simulink model "LQR_with_tracking"  (R2025b)
settings: Solver=ode45  StartTime=0.0  StopTime=Tend  MaxStep=1e-3  MinStep=1e-4  RelTol=1e-3
undefined symbols (not defined in the file): C, DiscIntNeverNeededParam, Kq, Kx, Ts
libraries: cstblocks x1
settings Model: Creator=davidecovolo  LastModifiedBy=davidecovolo
settings SolverCC: InitialStep=1e-4

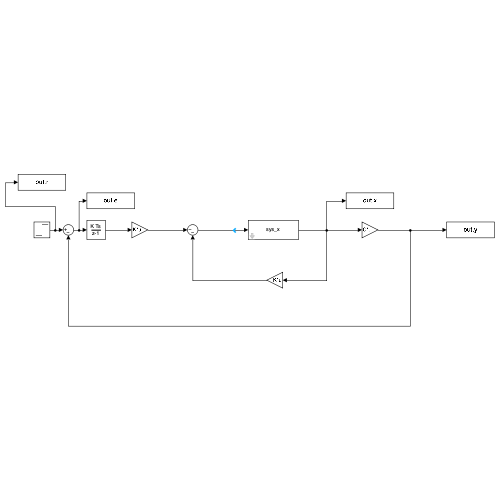
[thumbnail: Simulink's stored preview of the top-level diagram]
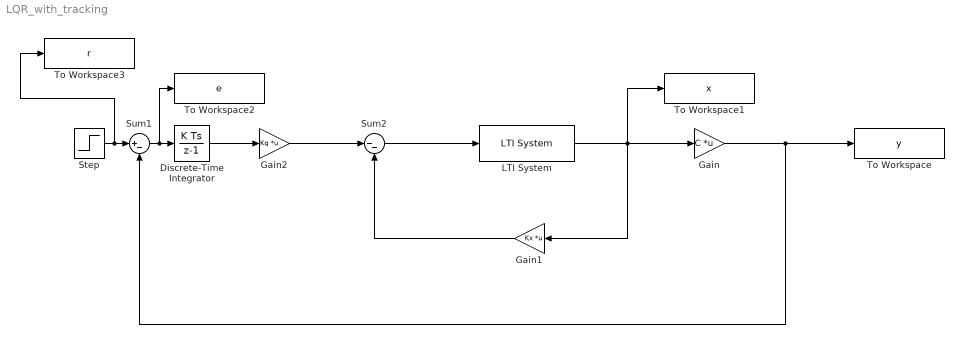
== system LQR_with_tracking ==
  Discrete-Time Integrator : DiscreteIntegrator  SampleTime=Ts  ICPrevOutput=DiscIntNeverNeededParam  ICPrevScaledInput=DiscIntNeverNeededParam
  Gain : Gain  Gain=C  Multiplication=Matrix(K*u)
  Gain1 : Gain  Gain=Kx  Multiplication=Matrix(K*u)
  Gain2 : Gain  Gain=Kq  Multiplication=Matrix(K*u)
  LTI System : cstblocks/LTI System  sys=sys_x  IC=x0  PadeOrder=0
  Step : Step  Time=0  SampleTime=0
  Sum1 : Sum  Inputs=|+-
  Sum2 : Sum  Inputs=|--
  To Workspace : ToWorkspace  VariableName=y  SaveFormat=Timeseries  SampleTime=Ts
  To Workspace1 : ToWorkspace  VariableName=x  SaveFormat=Timeseries  SampleTime=Ts
  To Workspace2 : ToWorkspace  VariableName=e  SaveFormat=Timeseries  SampleTime=Ts
  To Workspace3 : ToWorkspace  VariableName=r  SaveFormat=Timeseries  SampleTime=Ts
  wires:
  LTI System/1 -> To Workspace1/1, Gain1/1, Gain/1
  Gain2/1 -> Sum2/1
  Gain1/1 -> Sum2/2
  Discrete-Time Integrator/1 -> Gain2/1
  Step/1 -> To Workspace3/1, Sum1/1
  Sum1/1 -> To Workspace2/1, Discrete-Time Integrator/1
  Gain/1 -> Sum1/2, To Workspace/1
  Sum2/1 -> LTI System/1
